simulink model "a7DOF"  (R2021a)
settings: Solver=VariableStepAuto  StartTime=0.0  StopTime=10.0  RelTol=1e-3
(part 1 of 2)
settings Model: Creator=RickyFang  LastModifiedBy=RickyFang

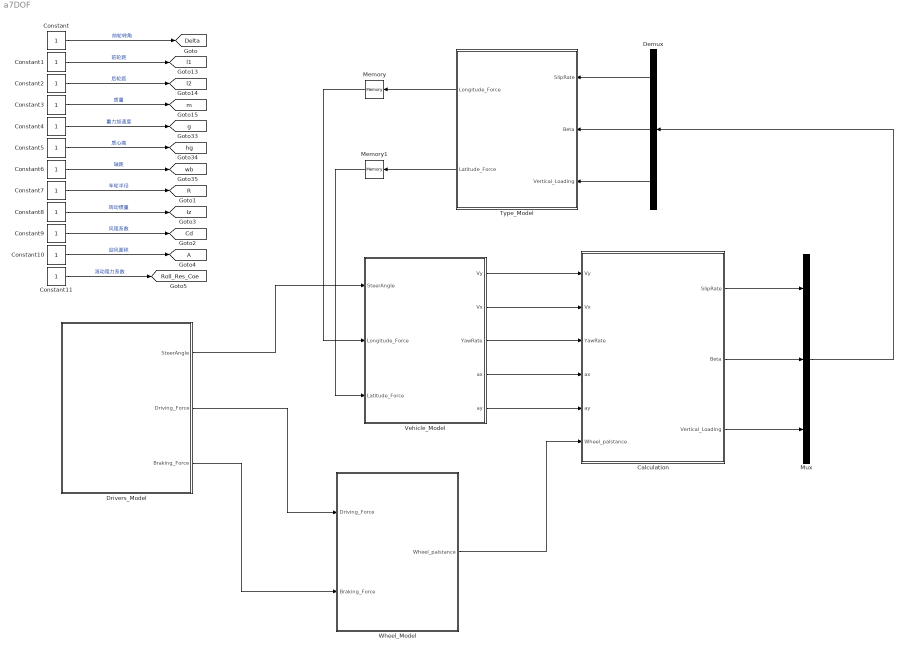
== system a7DOF ==
  Calculation : Subsystem
  Constant{,1..11} (12 alike) : Constant
  Demux : Demux  Outputs=3
  Drivers_Model : Subsystem
  Memory : Memory
  Memory1 : Memory
  Mux : Mux  Inputs=3
  Type_Model : Subsystem
  Vehicle_Model : Subsystem
  Wheel_Model : Subsystem
  tag scope: A=global, Cd=global, Delta=global, Iz=global, R=global, Roll_Res_Coe=global, g=global, hg=global, l1=global, l2=global, m=global, wb=global
  wires:
  Vehicle_Model/1(Vy) -> Calculation/1(Vy)
  Vehicle_Model/2(Vx) -> Calculation/2(Vx)
  Vehicle_Model/3(YawRate) -> Calculation/3(YawRate)
  Drivers_Model/1(SteerAngle) -> Vehicle_Model/1(SteerAngle)
  Drivers_Model/2(Driving_Force) -> Wheel_Model/1(Driving_Force)
  Drivers_Model/3(Braking_Force) -> Wheel_Model/2(Braking_Force)
  Calculation/2(Beta) -> Mux/2
  Calculation/1(SlipRate) -> Mux/1
  Demux/3 -> Type_Model/3(Vertical_Loading)
  Demux/2 -> Type_Model/2(Beta)
  Demux/1 -> Type_Model/1(SlipRate)
  Mux/1 -> Demux/1
  Calculation/3(Vertical_Loading) -> Mux/3
  Type_Model/2(Latitude_Force) -> Memory1/1
  Type_Model/1(Longitude_Force) -> Memory/1
  Memory/1 -> Vehicle_Model/2(Longitude_Force)
  Memory1/1 -> Vehicle_Model/3(Latitude_Force)
  Wheel_Model/1(Wheel_palstance) -> Calculation/6(Wheel_palstance)
  Vehicle_Model/4(ax) -> Calculation/4(ax)
  Vehicle_Model/5(ay) -> Calculation/5(ay)
  Constant/1 -> [Delta]  "前轮转角"
  Constant1/1 -> [l1]  "前轮距"
  Constant2/1 -> [l2]  "后轮距"
  Constant6/1 -> [wb]  "轴距"
  Constant5/1 -> [hg]  "质心高"
  Constant4/1 -> [g]  "重力加速度"
  Constant3/1 -> [m]  "质量"
  Constant7/1 -> [R]  "车轮半径"
  Constant8/1 -> [Iz]  "转动惯量"
  Constant9/1 -> [Cd]  "风阻系数"
  Constant10/1 -> [A]  "迎风面积"
  Constant11/1 -> [Roll_Res_Coe]  "滚动阻力系数"

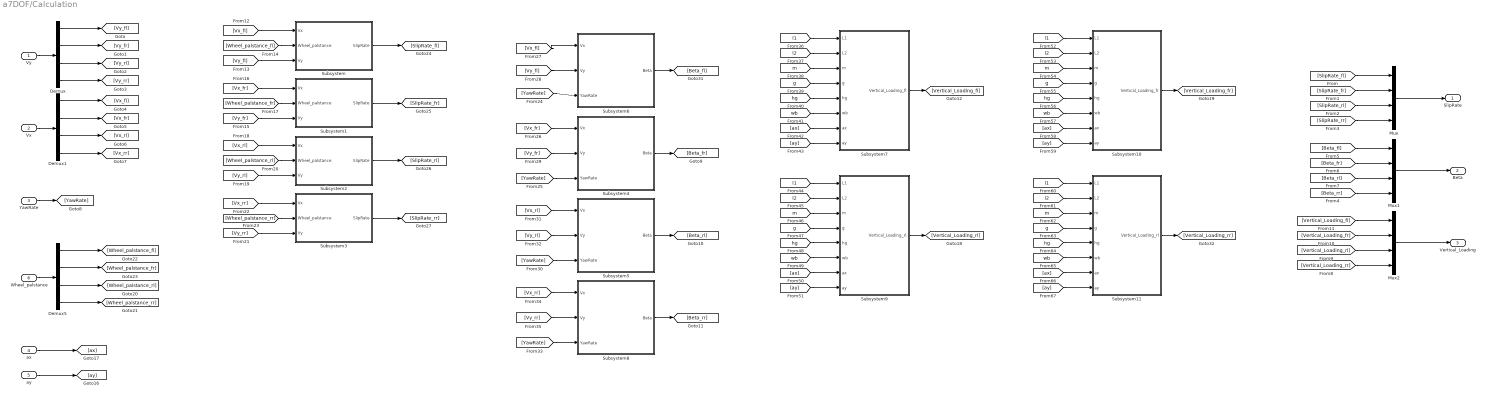
== system a7DOF/Calculation ==
  Vy : Inport
  Vx : Inport  Port=2
  YawRate : Inport  Port=3
  ax : Inport  Port=4
  ay : Inport  Port=5
  Wheel_palstance : Inport  Port=6
  Demux : Demux
  Demux1 : Demux
  Demux5 : Demux
  Mux : Mux
  Mux1 : Mux
  Mux2 : Mux
  Subsystem : Subsystem
  Subsystem1 : Subsystem
  Subsystem10 : Subsystem
  Subsystem11 : Subsystem
  Subsystem2 : Subsystem
  Subsystem3 : Subsystem
  Subsystem4 : Subsystem
  Subsystem5 : Subsystem
  Subsystem6 : Subsystem
  Subsystem7 : Subsystem
  Subsystem8 : Subsystem
  Subsystem9 : Subsystem
  SlipRate : Outport
  Beta : Outport  Port=2
  Vertical_Loading : Outport  Port=3
  wires:
  Vy/1 -> Demux/1
  Demux/1 -> [Vy_fl]
  Demux/2 -> [Vy_fr]
  Demux/3 -> [Vy_rl]
  Demux/4 -> [Vy_rr]
  Demux1/4 -> [Vx_rr]
  Demux1/3 -> [Vx_rl]
  Demux1/2 -> [Vx_fr]
  Demux1/1 -> [Vx_fl]
  Vx/1 -> Demux1/1
  YawRate/1 -> [YawRate]
  Demux5/4 -> [Wheel_palstance_rr]
  Demux5/3 -> [Wheel_palstance_rl]
  Demux5/2 -> [Wheel_palstance_fr]
  Demux5/1 -> [Wheel_palstance_fl]
  Wheel_palstance/1 -> Demux5/1
  Mux/1 -> SlipRate/1
  Mux1/1 -> Beta/1
  Mux2/1 -> Vertical_Loading/1
  [SlipRate_fl] -> Mux/1
  [SlipRate_fr] -> Mux/2
  [SlipRate_rl] -> Mux/3
  [SlipRate_rr] -> Mux/4
  [Beta_rr] -> Mux1/4
  [Beta_fl] -> Mux1/1
  [Beta_fr] -> Mux1/2
  [Beta_rl] -> Mux1/3
  [Vertical_Loading_rr] -> Mux2/4
  [Vertical_Loading_rl] -> Mux2/3
  [Vertical_Loading_fr] -> Mux2/2
  [Vertical_Loading_fl] -> Mux2/1
  [Vx_fl] -> Subsystem/1(Vx)
  [Vy_fl] -> Subsystem/3(Vy)
  [Wheel_palstance_fl] -> Subsystem/2(Wheel_palstance)
  [Vy_fr] -> Subsystem1/3(Vy)
  [Vx_fr] -> Subsystem1/1(Vx)
  [Wheel_palstance_fr] -> Subsystem1/2(Wheel_palstance)
  [Vx_rl] -> Subsystem2/1(Vx)
  [Vy_rl] -> Subsystem2/3(Vy)
  [Wheel_palstance_rl] -> Subsystem2/2(Wheel_palstance)
  [Vy_rr] -> Subsystem3/3(Vy)
  [Vx_rr] -> Subsystem3/1(Vx)
  [Wheel_palstance_rr] -> Subsystem3/2(Wheel_palstance)
  Subsystem/1(SlipRate) -> [SlipRate_fl]
  Subsystem1/1(SlipRate) -> [SlipRate_fr]
  Subsystem3/1(SlipRate) -> [SlipRate_rr]
  Subsystem2/1(SlipRate) -> [SlipRate_rl]
  [Vx_fl] -> Subsystem6/1(Vx)
  [Vy_fl] -> Subsystem6/2(Vy)
  Subsystem6/1(Beta) -> [Beta_fl]
  [l1] -> Subsystem7/1(L1)
  [l2] -> Subsystem7/2(L2)
  [m] -> Subsystem7/3(m)
  [g] -> Subsystem7/4(g)
  [hg] -> Subsystem7/5(hg)
  [wb] -> Subsystem7/6(wb)
  Subsystem7/1(Vertical_Loading_fl) -> [Vertical_Loading_fl]
  ay/1 -> [ay]
  ax/1 -> [ax]
  [ax] -> Subsystem7/7(ax)
  [ay] -> Subsystem7/8(ay)
  [ay] -> Subsystem9/8(ay)
  [ax] -> Subsystem9/7(ax)
  Subsystem9/1(Vertical_Loading_rl) -> [Vertical_Loading_rl]
  [wb] -> Subsystem9/6(wb)
  [hg] -> Subsystem9/5(hg)
  [g] -> Subsystem9/4(g)
  [m] -> Subsystem9/3(m)
  [l2] -> Subsystem9/2(L2)
  [l1] -> Subsystem9/1(L1)
  [l1] -> Subsystem10/1(L1)
  [l2] -> Subsystem10/2(L2)
  [m] -> Subsystem10/3(m)
  [g] -> Subsystem10/4(g)
  [hg] -> Subsystem10/5(hg)
  [wb] -> Subsystem10/6(wb)
  Subsystem10/1(Vertical_Loading_fr) -> [Vertical_Loading_fr]
  [ax] -> Subsystem10/7(ax)
  [ay] -> Subsystem10/8(ay)
  [ay] -> Subsystem11/8(ay)
  [ax] -> Subsystem11/7(ax)
  Subsystem11/1(Vertical_Loading_rl) -> [Vertical_Loading_rr]
  [wb] -> Subsystem11/6(wb)
  [hg] -> Subsystem11/5(hg)
  [g] -> Subsystem11/4(g)
  [m] -> Subsystem11/3(m)
  [l2] -> Subsystem11/2(L2)
  [l1] -> Subsystem11/1(L1)
  [YawRate] -> Subsystem6/3(YawRate)
  [YawRate] -> Subsystem4/3(YawRate)
  Subsystem4/1(Beta) -> [Beta_fr]
  [Vy_fr] -> Subsystem4/2(Vy)
  [Vx_fr] -> Subsystem4/1(Vx)
  [Vx_rl] -> Subsystem5/1(Vx)
  [Vy_rl] -> Subsystem5/2(Vy)
  Subsystem5/1(Beta) -> [Beta_rl]
  [YawRate] -> Subsystem5/3(YawRate)
  [YawRate] -> Subsystem8/3(YawRate)
  Subsystem8/1(Beta) -> [Beta_rr]
  [Vy_rr] -> Subsystem8/2(Vy)
  [Vx_rr] -> Subsystem8/1(Vx)

== system a7DOF/Drivers_Model ==
  SteerAngle : Outport
  Driving_Force : Outport  Port=2
  Braking_Force : Outport  Port=3
  wires:
  [Delta] -> SteerAngle/1

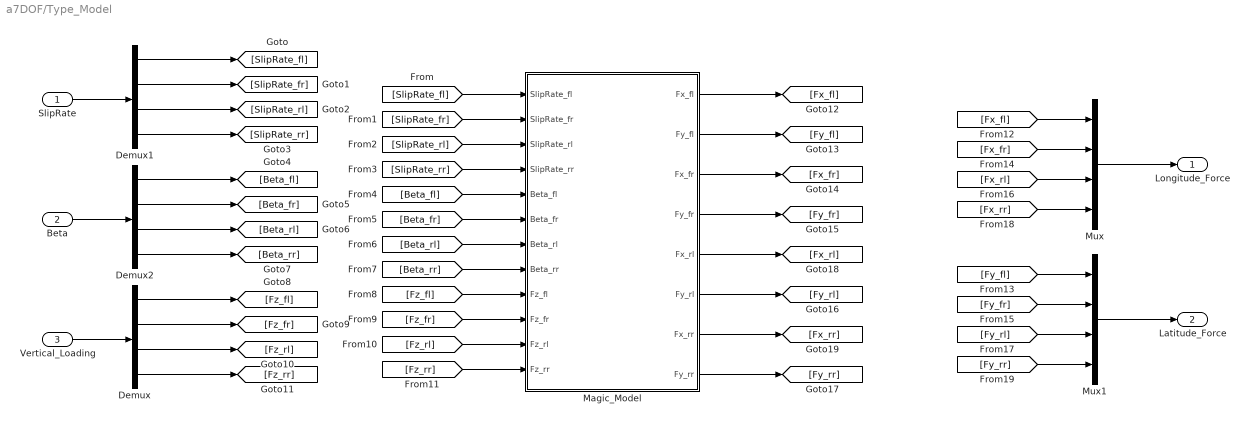
== system a7DOF/Type_Model ==
  SlipRate : Inport
  Beta : Inport  Port=2
  Vertical_Loading : Inport  Port=3
  Demux : Demux
  Demux1 : Demux
  Demux2 : Demux
  Magic_Model : Subsystem
  Mux : Mux
  Mux1 : Mux
  Longitude_Force : Outport
  Latitude_Force : Outport  Port=2
  wires:
  Vertical_Loading/1 -> Demux/1
  SlipRate/1 -> Demux1/1
  Beta/1 -> Demux2/1
  Demux1/1 -> [SlipRate_fl]
  Demux1/2 -> [SlipRate_fr]
  Demux1/3 -> [SlipRate_rl]
  Demux1/4 -> [SlipRate_rr]
  Demux2/4 -> [Beta_rr]
  Demux2/3 -> [Beta_rl]
  Demux2/2 -> [Beta_fr]
  Demux2/1 -> [Beta_fl]
  Demux/1 -> [Fz_fl]
  Demux/2 -> [Fz_fr]
  Demux/3 -> [Fz_rl]
  Demux/4 -> [Fz_rr]
  [SlipRate_fl] -> Magic_Model/1(SlipRate_fl)
  [SlipRate_fr] -> Magic_Model/2(SlipRate_fr)
  [SlipRate_rl] -> Magic_Model/3(SlipRate_rl)
  [SlipRate_rr] -> Magic_Model/4(SlipRate_rr)
  [Beta_fl] -> Magic_Model/5(Beta_fl)
  [Beta_fr] -> Magic_Model/6(Beta_fr)
  [Beta_rl] -> Magic_Model/7(Beta_rl)
  [Beta_rr] -> Magic_Model/8(Beta_rr)
  [Fz_fl] -> Magic_Model/9(Fz_fl)
  [Fz_fr] -> Magic_Model/10(Fz_fr)
  [Fz_rl] -> Magic_Model/11(Fz_rl)
  [Fz_rr] -> Magic_Model/12(Fz_rr)
  Magic_Model/1(Fx_fl) -> [Fx_fl]
  Magic_Model/2(Fy_fl) -> [Fy_fl]
  Magic_Model/3(Fx_fr) -> [Fx_fr]
  Magic_Model/4(Fy_fr) -> [Fy_fr]
  Magic_Model/6(Fy_rl) -> [Fy_rl]
  Magic_Model/8(Fy_rr) -> [Fy_rr]
  Magic_Model/5(Fx_rl) -> [Fx_rl]
  Magic_Model/7(Fx_rr) -> [Fx_rr]
  [Fx_fl] -> Mux/1
  [Fx_rr] -> Mux/4
  [Fx_fr] -> Mux/2
  [Fx_rl] -> Mux/3
  Mux/1 -> Longitude_Force/1
  [Fy_fl] -> Mux1/1
  [Fy_fr] -> Mux1/2
  [Fy_rr] -> Mux1/4
  [Fy_rl] -> Mux1/3
  Mux1/1 -> Latitude_Force/1

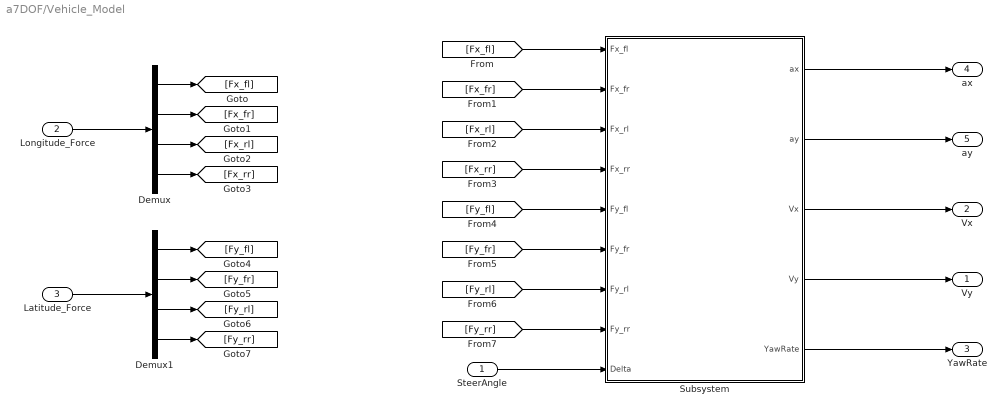
== system a7DOF/Vehicle_Model ==
  SteerAngle : Inport
  Longitude_Force : Inport  Port=2
  Latitude_Force : Inport  Port=3
  Demux : Demux
  Demux1 : Demux
  Subsystem : Subsystem
  Vy : Outport
  Vx : Outport  Port=2
  YawRate : Outport  Port=3
  ax : Outport  Port=4
  ay : Outport  Port=5
  wires:
  Longitude_Force/1 -> Demux/1
  Latitude_Force/1 -> Demux1/1
  Demux/1 -> [Fx_fl]
  Demux/2 -> [Fx_fr]
  Demux/3 -> [Fx_rl]
  Demux/4 -> [Fx_rr]
  Demux1/1 -> [Fy_fl]
  Demux1/2 -> [Fy_fr]
  Demux1/3 -> [Fy_rl]
  Demux1/4 -> [Fy_rr]
  [Fx_fl] -> Subsystem/1(Fx_fl)
  [Fx_fr] -> Subsystem/2(Fx_fr)
  [Fx_rl] -> Subsystem/3(Fx_rl)
  [Fx_rr] -> Subsystem/4(Fx_rr)
  [Fy_rr] -> Subsystem/8(Fy_rr)
  [Fy_rl] -> Subsystem/7(Fy_rl)
  [Fy_fr] -> Subsystem/6(Fy_fr)
  [Fy_fl] -> Subsystem/5(Fy_fl)
  SteerAngle/1 -> Subsystem/9(Delta)
  Subsystem/2(ay) -> ay/1
  Subsystem/4(Vy) -> Vy/1
  Subsystem/3(Vx) -> Vx/1
  Subsystem/1(ax) -> ax/1
  Subsystem/5(YawRate) -> YawRate/1

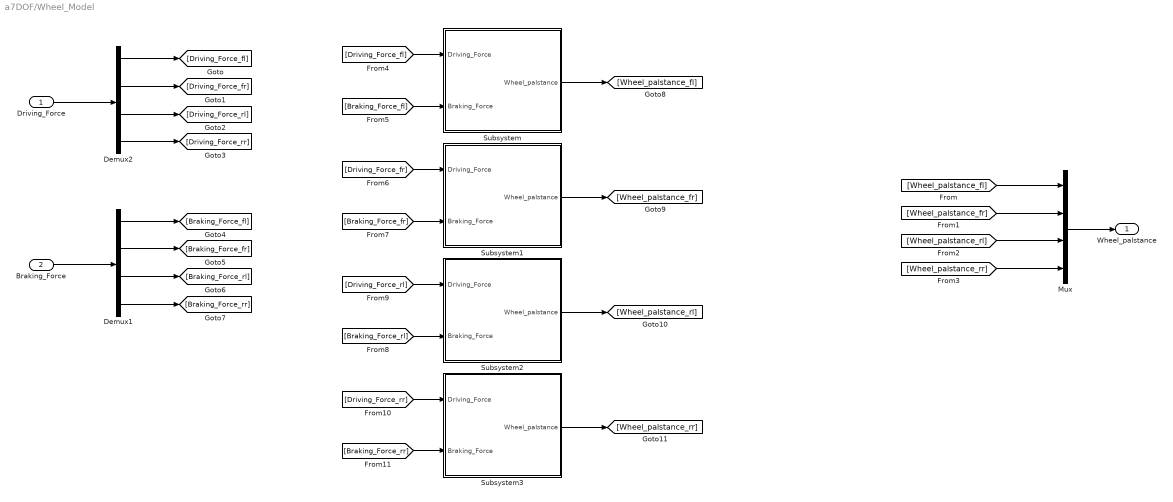
== system a7DOF/Wheel_Model ==
  Driving_Force : Inport
  Braking_Force : Inport  Port=2
  Demux1 : Demux
  Demux2 : Demux
  Mux : Mux
  Subsystem : Subsystem
  Subsystem1 : Subsystem
  Subsystem2 : Subsystem
  Subsystem3 : Subsystem
  Wheel_palstance : Outport
  wires:
  Driving_Force/1 -> Demux2/1
  Braking_Force/1 -> Demux1/1
  Demux2/1 -> [Driving_Force_fl]
  Demux2/2 -> [Driving_Force_fr]
  Demux2/3 -> [Driving_Force_rl]
  Demux2/4 -> [Driving_Force_rr]
  Demux1/1 -> [Braking_Force_fl]
  Demux1/2 -> [Braking_Force_fr]
  Demux1/3 -> [Braking_Force_rl]
  Demux1/4 -> [Braking_Force_rr]
  Mux/1 -> Wheel_palstance/1
  [Wheel_palstance_fr] -> Mux/2
  [Wheel_palstance_fl] -> Mux/1
  [Wheel_palstance_rl] -> Mux/3
  [Wheel_palstance_rr] -> Mux/4
  [Driving_Force_fl] -> Subsystem/1(Driving_Force)
  [Braking_Force_fl] -> Subsystem/2(Braking_Force)
  Subsystem/1(Wheel_palstance) -> [Wheel_palstance_fl]
  Subsystem1/1(Wheel_palstance) -> [Wheel_palstance_fr]
  [Driving_Force_fr] -> Subsystem1/1(Driving_Force)
  [Braking_Force_fr] -> Subsystem1/2(Braking_Force)
  [Driving_Force_rl] -> Subsystem2/1(Driving_Force)
  [Braking_Force_rl] -> Subsystem2/2(Braking_Force)
  Subsystem2/1(Wheel_palstance) -> [Wheel_palstance_rl]
  Subsystem3/1(Wheel_palstance) -> [Wheel_palstance_rr]
  [Braking_Force_rr] -> Subsystem3/2(Braking_Force)
  [Driving_Force_rr] -> Subsystem3/1(Driving_Force)

== system a7DOF/Calculation/Subsystem ==
  Vx : Inport
  Wheel_palstance : Inport  Port=2
  Vy : Inport  Port=3
  Abs : Abs
  Add : Sum
  Add1 : Sum  Inputs=+-
  Cos : Trigonometry  Operator=cos
  Cos1 : Trigonometry
  Divide : Product  Inputs=*/
  Max : MinMax  Function=max  Inputs=2
  Product : Product
  Product1 : Product
  Product2 : Product
  SlipRate : Outport
  wires:
  Wheel_palstance/1 -> Product/1
  [R] -> Product/2
  Divide/1 -> SlipRate/1
  [Delta] -> Cos/1
  Cos/1 -> Product1/1
  Vx/1 -> Product1/2
  Product1/1 -> Add/2
  Cos1/1 -> Product2/1
  [Delta] -> Cos1/1
  Vy/1 -> Product2/2
  Product2/1 -> Add/1
  Add/1 -> Max/1, Add1/1
  Product/1 -> Max/2, Add1/2
  Add1/1 -> Abs/1
  Abs/1 -> Divide/1
  Max/1 -> Divide/2

== system a7DOF/Calculation/Subsystem1 ==
  Vx : Inport
  Wheel_palstance : Inport  Port=2
  Vy : Inport  Port=3
  Abs : Abs
  Add : Sum
  Add1 : Sum  Inputs=+-
  Cos : Trigonometry  Operator=cos
  Cos1 : Trigonometry
  Divide : Product  Inputs=*/
  Max : MinMax  Function=max  Inputs=2
  Product : Product
  Product1 : Product
  Product2 : Product
  SlipRate : Outport
  wires:
  Max/1 -> Divide/2
  Abs/1 -> Divide/1
  Add1/1 -> Abs/1
  Product/1 -> Add1/2, Max/2
  Add/1 -> Add1/1, Max/1
  Product2/1 -> Add/1
  Vy/1 -> Product2/2
  [Delta] -> Cos1/1
  Cos1/1 -> Product2/1
  Product1/1 -> Add/2
  Vx/1 -> Product1/2
  Cos/1 -> Product1/1
  [Delta] -> Cos/1
  Divide/1 -> SlipRate/1
  [R] -> Product/2
  Wheel_palstance/1 -> Product/1

== system a7DOF/Calculation/Subsystem10 ==
  L1 : Inport
  L2 : Inport  Port=2
  m : Inport  Port=3
  g : Inport  Port=4
  hg : Inport  Port=5
  wb : Inport  Port=6
  ax : Inport  Port=7
  ay : Inport  Port=8
  Add : Sum  Inputs=+-+
  Subsystem : Subsystem
  Subsystem1 : Subsystem
  Subsystem2 : Subsystem
  Vertical_Loading_fr : Outport
  wires:
  m/1 -> Subsystem2/4(In4), Subsystem1/3(In3), Subsystem/3(In3)
  g/1 -> Subsystem/4(In4)
  hg/1 -> Subsystem2/5(In5), Subsystem1/4(In4)
  ax/1 -> Subsystem1/5(In5)
  L1/1 -> Subsystem2/1(In1), Subsystem1/1(In1), Subsystem/1(In1)
  L2/1 -> Subsystem2/2(In2), Subsystem2/3(In3), Subsystem1/2(In2), Subsystem/2(In2)
  wb/1 -> Subsystem2/6(In6)
  ay/1 -> Subsystem2/7(In7)
  Subsystem1/1(Out1) -> Add/2
  Subsystem/1(Out1) -> Add/1
  Subsystem2/1(Out1) -> Add/3
  Add/1 -> Vertical_Loading_fr/1

== system a7DOF/Calculation/Subsystem11 ==
  L1 : Inport
  L2 : Inport  Port=2
  m : Inport  Port=3
  g : Inport  Port=4
  hg : Inport  Port=5
  wb : Inport  Port=6
  ax : Inport  Port=7
  ay : Inport  Port=8
  Add : Sum  Inputs=+++
  Subsystem : Subsystem
  Subsystem1 : Subsystem
  Subsystem2 : Subsystem
  Vertical_Loading_rl : Outport
  wires:
  m/1 -> Subsystem2/4(In4), Subsystem1/3(In3), Subsystem/3(In3)
  g/1 -> Subsystem/4(In4)
  hg/1 -> Subsystem2/5(In5), Subsystem1/4(In4)
  ax/1 -> Subsystem1/5(In5)
  L1/1 -> Subsystem2/1(In1), Subsystem1/1(In1), Subsystem/1(In1)
  L2/1 -> Subsystem2/2(In2), Subsystem2/3(In3), Subsystem1/2(In2), Subsystem/2(In2)
  wb/1 -> Subsystem2/6(In6)
  ay/1 -> Subsystem2/7(In7)
  Subsystem1/1(Out1) -> Add/2
  Subsystem/1(Out1) -> Add/1
  Subsystem2/1(Out1) -> Add/3
  Add/1 -> Vertical_Loading_rl/1

== system a7DOF/Calculation/Subsystem2 ==
  Vx : Inport
  Wheel_palstance : Inport  Port=2
  Vy : Inport  Port=3
  Abs : Abs
  Add : Sum
  Add1 : Sum  Inputs=+-
  Cos : Trigonometry  Operator=cos
  Cos1 : Trigonometry
  Divide : Product  Inputs=*/
  Max : MinMax  Function=max  Inputs=2
  Product : Product
  Product1 : Product
  Product2 : Product
  SlipRate : Outport
  wires:
  Wheel_palstance/1 -> Product/1
  [R] -> Product/2
  Divide/1 -> SlipRate/1
  [Delta] -> Cos/1
  Cos/1 -> Product1/1
  Vx/1 -> Product1/2
  Product1/1 -> Add/2
  Cos1/1 -> Product2/1
  [Delta] -> Cos1/1
  Vy/1 -> Product2/2
  Product2/1 -> Add/1
  Add/1 -> Max/1, Add1/1
  Product/1 -> Max/2, Add1/2
  Add1/1 -> Abs/1
  Abs/1 -> Divide/1
  Max/1 -> Divide/2

== system a7DOF/Calculation/Subsystem3 ==
  Vx : Inport
  Wheel_palstance : Inport  Port=2
  Vy : Inport  Port=3
  Abs : Abs
  Add : Sum
  Add1 : Sum  Inputs=+-
  Cos : Trigonometry  Operator=cos
  Cos1 : Trigonometry
  Divide : Product  Inputs=*/
  Max : MinMax  Function=max  Inputs=2
  Product : Product
  Product1 : Product
  Product2 : Product
  SlipRate : Outport
  wires:
  Max/1 -> Divide/2
  Abs/1 -> Divide/1
  Add1/1 -> Abs/1
  Product/1 -> Add1/2, Max/2
  Add/1 -> Add1/1, Max/1
  Product2/1 -> Add/1
  Vy/1 -> Product2/2
  [Delta] -> Cos1/1
  Cos1/1 -> Product2/1
  Product1/1 -> Add/2
  Vx/1 -> Product1/2
  Cos/1 -> Product1/1
  [Delta] -> Cos/1
  Divide/1 -> SlipRate/1
  [R] -> Product/2
  Wheel_palstance/1 -> Product/1

== system a7DOF/Calculation/Subsystem4 ==
  Vx : Inport
  Vy : Inport  Port=2
  YawRate : Inport  Port=3
  Add : Sum
  Add1 : Sum
  Add2 : Sum  Inputs=+-
  Atan : Trigonometry  Operator=atan
  Divide : Product  Inputs=/*
  Gain : Gain  Gain=0.5
  Product : Product
  Product1 : Product
  YawRate1 : InportShadow  Port=3
  Beta : Outport
  wires:
  Add2/1 -> Beta/1
  Atan/1 -> Add2/2
  [Delta] -> Add2/1
  Divide/1 -> Atan/1
  Add/1 -> Divide/2
  Add1/1 -> Divide/1
  Product1/1 -> Add1/2
  Vx/1 -> Add1/1
  Gain/1 -> Product1/2
  [wb] -> Gain/1
  YawRate1/1 -> Product1/1
  Product/1 -> Add/2
  YawRate/1 -> Product/2
  [l1] -> Product/1
  Vy/1 -> Add/1

== system a7DOF/Calculation/Subsystem5 ==
  Vx : Inport
  Vy : Inport  Port=2
  YawRate : Inport  Port=3
  Add : Sum  Inputs=+-
  Add1 : Sum  Inputs=+-
  Atan : Trigonometry  Operator=atan
  Divide : Product  Inputs=/*
  Gain : Gain  Gain=0.5
  Gain1 : Gain  Gain=-1
  Product : Product
  Product1 : Product
  YawRate1 : InportShadow  Port=3
  Beta : Outport
  wires:
  Vy/1 -> Add/1
  [l2] -> Product/1
  YawRate/1 -> Product/2
  Product/1 -> Add/2
  YawRate1/1 -> Product1/1
  [wb] -> Gain/1
  Gain/1 -> Product1/2
  Vx/1 -> Add1/1
  Product1/1 -> Add1/2
  Add1/1 -> Divide/1
  Add/1 -> Divide/2
  Divide/1 -> Atan/1
  Gain1/1 -> Beta/1
  Atan/1 -> Gain1/1

== system a7DOF/Calculation/Subsystem6 ==
  Vx : Inport
  Vy : Inport  Port=2
  YawRate : Inport  Port=3
  Add : Sum
  Add1 : Sum  Inputs=+-
  Add2 : Sum  Inputs=+-
  Atan : Trigonometry  Operator=atan
  Divide : Product  Inputs=/*
  Gain : Gain  Gain=0.5
  Product : Product
  Product1 : Product
  YawRate1 : InportShadow  Port=3
  Beta : Outport
  wires:
  Vy/1 -> Add/1
  [l1] -> Product/1
  YawRate/1 -> Product/2
  Product/1 -> Add/2
  YawRate1/1 -> Product1/1
  [wb] -> Gain/1
  Gain/1 -> Product1/2
  Vx/1 -> Add1/1
  Product1/1 -> Add1/2
  Add1/1 -> Divide/1
  Add/1 -> Divide/2
  Divide/1 -> Atan/1
  [Delta] -> Add2/1
  Atan/1 -> Add2/2
  Add2/1 -> Beta/1

== system a7DOF/Calculation/Subsystem7 ==
  L1 : Inport
  L2 : Inport  Port=2
  m : Inport  Port=3
  g : Inport  Port=4
  hg : Inport  Port=5
  wb : Inport  Port=6
  ax : Inport  Port=7
  ay : Inport  Port=8
  Add : Sum  Inputs=+--
  Subsystem : Subsystem
  Subsystem1 : Subsystem
  Subsystem2 : Subsystem
  Vertical_Loading_fl : Outport
  wires:
  m/1 -> Subsystem2/4(In4), Subsystem1/3(In3), Subsystem/3(In3)
  g/1 -> Subsystem/4(In4)
  hg/1 -> Subsystem2/5(In5), Subsystem1/4(In4)
  ax/1 -> Subsystem1/5(In5)
  L1/1 -> Subsystem2/1(In1), Subsystem1/1(In1), Subsystem/1(In1)
  L2/1 -> Subsystem2/2(In2), Subsystem2/3(In3), Subsystem1/2(In2), Subsystem/2(In2)
  wb/1 -> Subsystem2/6(In6)
  ay/1 -> Subsystem2/7(In7)
  Subsystem1/1(Out1) -> Add/2
  Subsystem/1(Out1) -> Add/1
  Subsystem2/1(Out1) -> Add/3
  Add/1 -> Vertical_Loading_fl/1

== system a7DOF/Calculation/Subsystem8 ==
  Vx : Inport
  Vy : Inport  Port=2
  YawRate : Inport  Port=3
  Add : Sum  Inputs=+-
  Add1 : Sum
  Atan : Trigonometry  Operator=atan
  Divide : Product  Inputs=/*
  Gain : Gain  Gain=0.5
  Gain1 : Gain  Gain=-1
  Product : Product
  Product1 : Product
  YawRate1 : InportShadow  Port=3
  Beta : Outport
  wires:
  Atan/1 -> Gain1/1
  Gain1/1 -> Beta/1
  Divide/1 -> Atan/1
  Add/1 -> Divide/2
  Add1/1 -> Divide/1
  Product1/1 -> Add1/2
  Vx/1 -> Add1/1
  Gain/1 -> Product1/2
  [wb] -> Gain/1
  YawRate1/1 -> Product1/1
  Product/1 -> Add/2
  YawRate/1 -> Product/2
  [l2] -> Product/1
  Vy/1 -> Add/1

== system a7DOF/Calculation/Subsystem9 ==
  L1 : Inport
  L2 : Inport  Port=2
  m : Inport  Port=3
  g : Inport  Port=4
  hg : Inport  Port=5
  wb : Inport  Port=6
  ax : Inport  Port=7
  ay : Inport  Port=8
  Add : Sum  Inputs=++-
  Subsystem : Subsystem
  Subsystem1 : Subsystem
  Subsystem2 : Subsystem
  Vertical_Loading_rl : Outport
  wires:
  Add/1 -> Vertical_Loading_rl/1
  Subsystem2/1(Out1) -> Add/3
  Subsystem/1(Out1) -> Add/1
  Subsystem1/1(Out1) -> Add/2
  ay/1 -> Subsystem2/7(In7)
  wb/1 -> Subsystem2/6(In6)
  L2/1 -> Subsystem/2(In2), Subsystem1/2(In2), Subsystem2/3(In3), Subsystem2/2(In2)
  L1/1 -> Subsystem/1(In1), Subsystem1/1(In1), Subsystem2/1(In1)
  ax/1 -> Subsystem1/5(In5)
  hg/1 -> Subsystem1/4(In4), Subsystem2/5(In5)
  g/1 -> Subsystem/4(In4)
  m/1 -> Subsystem/3(In3), Subsystem1/3(In3), Subsystem2/4(In4)

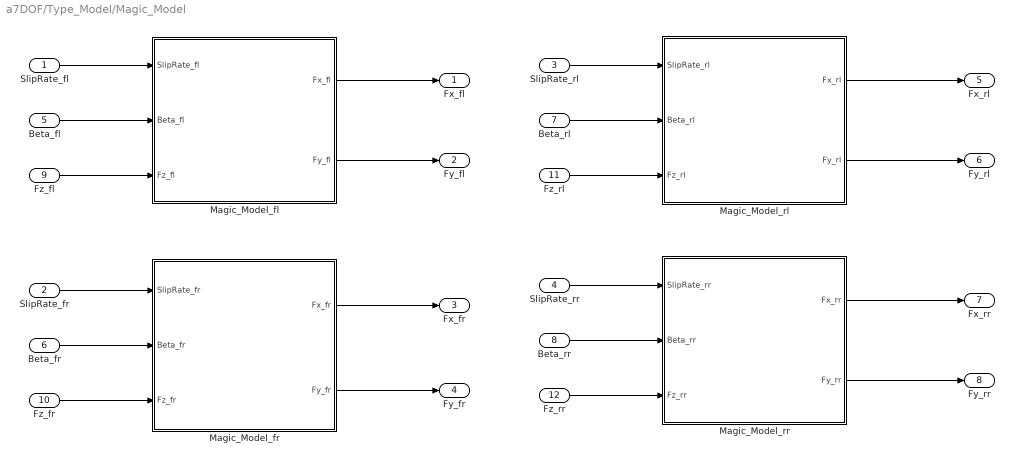
== system a7DOF/Type_Model/Magic_Model ==
  SlipRate_fl : Inport
  SlipRate_fr : Inport  Port=2
  SlipRate_rl : Inport  Port=3
  SlipRate_rr : Inport  Port=4
  Beta_fl : Inport  Port=5
  Beta_fr : Inport  Port=6
  Beta_rl : Inport  Port=7
  Beta_rr : Inport  Port=8
  Fz_fl : Inport  Port=9
  Fz_fr : Inport  Port=10
  Fz_rl : Inport  Port=11
  Fz_rr : Inport  Port=12
  Magic_Model_fl : Subsystem
  Magic_Model_fr : Subsystem
  Magic_Model_rl : Subsystem
  Magic_Model_rr : Subsystem
  Fx_fl : Outport
  Fy_fl : Outport  Port=2
  Fx_fr : Outport  Port=3
  Fy_fr : Outport  Port=4
  Fx_rl : Outport  Port=5
  Fy_rl : Outport  Port=6
  Fx_rr : Outport  Port=7
  Fy_rr : Outport  Port=8
  wires:
  SlipRate_fl/1 -> Magic_Model_fl/1(SlipRate_fl)
  Beta_fl/1 -> Magic_Model_fl/2(Beta_fl)
  Fz_fl/1 -> Magic_Model_fl/3(Fz_fl)
  Magic_Model_fl/1(Fx_fl) -> Fx_fl/1
  Magic_Model_fl/2(Fy_fl) -> Fy_fl/1
  SlipRate_fr/1 -> Magic_Model_fr/1(SlipRate_fr)
  Beta_fr/1 -> Magic_Model_fr/2(Beta_fr)
  Fz_fr/1 -> Magic_Model_fr/3(Fz_fr)
  Magic_Model_fr/1(Fx_fr) -> Fx_fr/1
  Magic_Model_fr/2(Fy_fr) -> Fy_fr/1
  SlipRate_rl/1 -> Magic_Model_rl/1(SlipRate_rl)
  Beta_rl/1 -> Magic_Model_rl/2(Beta_rl)
  Fz_rl/1 -> Magic_Model_rl/3(Fz_rl)
  Magic_Model_rl/1(Fx_rl) -> Fx_rl/1
  Magic_Model_rl/2(Fy_rl) -> Fy_rl/1
  SlipRate_rr/1 -> Magic_Model_rr/1(SlipRate_rr)
  Beta_rr/1 -> Magic_Model_rr/2(Beta_rr)
  Fz_rr/1 -> Magic_Model_rr/3(Fz_rr)
  Magic_Model_rr/1(Fx_rr) -> Fx_rr/1
  Magic_Model_rr/2(Fy_rr) -> Fy_rr/1

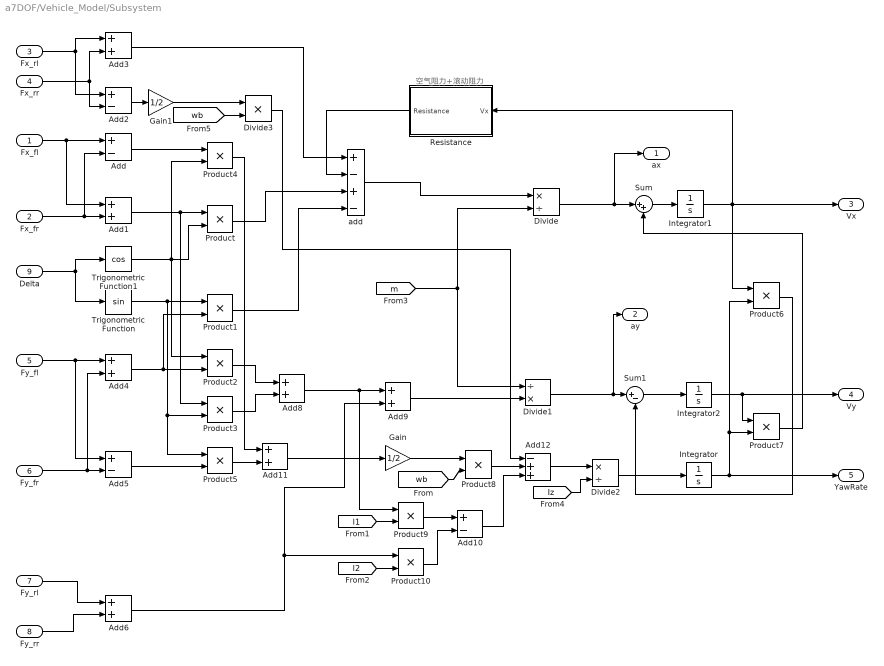
== system a7DOF/Vehicle_Model/Subsystem ==
  note: 空气阻力+滚动阻力
  Fx_fl : Inport
  Fx_fr : Inport  Port=2
  Fx_rl : Inport  Port=3
  Fx_rr : Inport  Port=4
  Fy_fl : Inport  Port=5
  Fy_fr : Inport  Port=6
  Fy_rl : Inport  Port=7
  Fy_rr : Inport  Port=8
  Delta : Inport  Port=9
  Add{,2,5,10} (4 alike) : Sum  Inputs=+-
  Add{1,3..4,6,8..9,11} (7 alike) : Sum
  Add12 : Sum  Inputs=-++
  Divide : Product  Inputs=*/
  Divide1 : Product  Inputs=/*
  Divide2 : Product  Inputs=*/
  Divide3 : Product  Inputs=**
  Gain : Gain  Gain=1/2
  Gain1 : Gain  Gain=1/2
  Integrator : Integrator
  Integrator1 : Integrator  InitialCondition=eps  UpperSaturationLimit=35  LowerSaturationLimit=0
  Integrator2 : Integrator
  Product{,1..7} (8 alike) : Product  RndMeth=Zero
  Product10 : Product
  Product8 : Product
  Product9 : Product
  Resistance : Subsystem
  Sum : Sum  Inputs=|++
  Sum1 : Sum  Inputs=|+-
  Trigonometric Function : Trigonometry
  Trigonometric Function1 : Trigonometry  Operator=cos
  add : Sum  Inputs=+-+-
  ax : Outport
  ay : Outport  Port=2
  Vx : Outport  Port=3
  Vy : Outport  Port=4
  YawRate : Outport  Port=5
  wires:
  Sum1/1 -> Integrator2/1
  Add9/1 -> Divide1/2
  Fx_fr/1 -> Add/2, Add1/2
  Sum/1 -> Integrator1/1
  Resistance/1(Resistance) -> add/2
  add/1 -> Divide/1
  Product2/1 -> Add8/1
  Add2/1 -> Gain1/1
  Product8/1 -> Add12/2
  Add8/1 -> Product9/1, Add9/1
  Add/1 -> Product4/1
  Integrator2/1 -> Product7/1, Vy/1
  Product3/1 -> Add8/2
  Product5/1 -> Add11/2
  Add6/1 -> Product10/1, Add9/2
  [m] -> Divide1/1, Divide/2
  Fx_rr/1 -> Add3/2, Add2/2
  Add4/1 -> Product1/2, Product2/2
  Product9/1 -> Add10/1
  Fy_fl/1 -> Add4/1, Add5/1
  Trigonometric Function/1 -> Product1/1, Product3/2, Product5/1
  Divide/1 -> Sum/1, ax/1
  Add3/1 -> add/1
  Fx_fl/1 -> Add/1, Add1/1
  Divide2/1 -> Integrator/1
  Add1/1 -> Product/1, Product3/1
  Integrator1/1 -> Product6/1, Vx/1, Resistance/1("Vx ")
  Delta/1 -> Trigonometric Function/1, Trigonometric Function1/1
  Fx_rl/1 -> Add2/1, Add3/1
  Fy_rl/1 -> Add6/1
  Trigonometric Function1/1 -> Product/2, Product2/1, Product4/2
  Product1/1 -> add/4
  Product10/1 -> Add10/2
  Product/1 -> add/3
  Add10/1 -> Add12/3
  Fy_rr/1 -> Add6/2
  Product4/1 -> Add11/1
  Product6/1 -> Sum1/2
  Divide1/1 -> Sum1/1, ay/1
  Product7/1 -> Sum/2
  Add12/1 -> Divide2/1
  Fy_fr/1 -> Add5/2, Add4/2
  Integrator/1 -> Product6/2, Product7/2, YawRate/1
  Add5/1 -> Product5/2
  [wb] -> Product8/2
  Add11/1 -> Gain/1
  Gain/1 -> Product8/1
  [l1] -> Product9/2
  [l2] -> Product10/2
  [Iz] -> Divide2/2
  Divide3/1 -> Add12/1
  Gain1/1 -> Divide3/1
  [wb] -> Divide3/2

== system a7DOF/Wheel_Model/Subsystem ==
  Driving_Force : Inport
  Braking_Force : Inport  Port=2
  Add : Sum  Inputs=+-
  Divide : Product  Inputs=*//
  Integrator : Integrator
  Wheel_palstance : Outport
  wires:
  Divide/1 -> Integrator/1
  Braking_Force/1 -> Add/2
  Add/1 -> Divide/1
  [m] -> Divide/3
  [R] -> Divide/2
  Driving_Force/1 -> Add/1
  Integrator/1 -> Wheel_palstance/1

== system a7DOF/Wheel_Model/Subsystem1 ==
  Driving_Force : Inport
  Braking_Force : Inport  Port=2
  Add : Sum  Inputs=+-
  Divide : Product  Inputs=*//
  Integrator : Integrator
  Wheel_palstance : Outport
  wires:
  Integrator/1 -> Wheel_palstance/1
  Driving_Force/1 -> Add/1
  [R] -> Divide/2
  [m] -> Divide/3
  Add/1 -> Divide/1
  Braking_Force/1 -> Add/2
  Divide/1 -> Integrator/1

== system a7DOF/Wheel_Model/Subsystem2 ==
  Driving_Force : Inport
  Braking_Force : Inport  Port=2
  Add : Sum  Inputs=+-
  Divide : Product  Inputs=*//
  Integrator : Integrator
  Wheel_palstance : Outport
  wires:
  Divide/1 -> Integrator/1
  Braking_Force/1 -> Add/2
  Add/1 -> Divide/1
  [m] -> Divide/3
  [R] -> Divide/2
  Driving_Force/1 -> Add/1
  Integrator/1 -> Wheel_palstance/1

== system a7DOF/Wheel_Model/Subsystem3 ==
  Driving_Force : Inport
  Braking_Force : Inport  Port=2
  Add : Sum  Inputs=+-
  Divide : Product  Inputs=*//
  Integrator : Integrator
  Wheel_palstance : Outport
  wires:
  Integrator/1 -> Wheel_palstance/1
  Driving_Force/1 -> Add/1
  [R] -> Divide/2
  [m] -> Divide/3
  Add/1 -> Divide/1
  Braking_Force/1 -> Add/2
  Divide/1 -> Integrator/1

== system a7DOF/Calculation/Subsystem10/Subsystem ==
  In1 : Inport
  In2 : Inport  Port=2
  In3 : Inport  Port=3
  In4 : Inport  Port=4
  Add : Sum
  Divide : Product  Inputs=***/
  Gain : Gain  Gain=2
  Out1 : Outport
  wires:
  In1/1 -> Add/1
  Add/1 -> Gain/1
  In2/1 -> Divide/1, Add/2
  Gain/1 -> Divide/4
  In3/1 -> Divide/2
  Divide/1 -> Out1/1
  In4/1 -> Divide/3

== system a7DOF/Calculation/Subsystem10/Subsystem1 ==
  In1 : Inport
  In2 : Inport  Port=2
  In3 : Inport  Port=3
  In4 : Inport  Port=4
  In5 : Inport  Port=5
  Add : Sum
  Divide : Product  Inputs=***/
  Gain : Gain  Gain=2
  Out1 : Outport
  wires:
  Divide/1 -> Out1/1
  In4/1 -> Divide/3
  Gain/1 -> Divide/4
  In3/1 -> Divide/1
  In1/1 -> Add/1
  Add/1 -> Gain/1
  In5/1 -> Divide/2
  In2/1 -> Add/2

== system a7DOF/Calculation/Subsystem10/Subsystem2 ==
  In1 : Inport
  In2 : Inport  Port=2
  In3 : Inport  Port=3
  In4 : Inport  Port=4
  In5 : Inport  Port=5
  In6 : Inport  Port=6
  In7 : Inport  Port=7
  Add : Sum
  Divide : Product  Inputs=****//
  Gain : Gain  Gain=2
  Out1 : Outport
  wires:
  In6/1 -> Divide/5
  In3/1 -> Divide/4
  Add/1 -> Gain/1
  Divide/1 -> Out1/1
  In2/1 -> Add/2
  In1/1 -> Add/1
  Gain/1 -> Divide/6
  In4/1 -> Divide/1
  In7/1 -> Divide/2
  In5/1 -> Divide/3

== system a7DOF/Calculation/Subsystem11/Subsystem ==
  In1 : Inport
  In2 : Inport  Port=2
  In3 : Inport  Port=3
  In4 : Inport  Port=4
  Add : Sum
  Divide : Product  Inputs=***/
  Gain : Gain  Gain=2
  Out1 : Outport
  wires:
  In2/1 -> Add/1
  Add/1 -> Gain/1
  In1/1 -> Divide/1, Add/2
  Gain/1 -> Divide/4
  In3/1 -> Divide/2
  Divide/1 -> Out1/1
  In4/1 -> Divide/3

== system a7DOF/Calculation/Subsystem11/Subsystem1 ==
  In1 : Inport
  In2 : Inport  Port=2
  In3 : Inport  Port=3
  In4 : Inport  Port=4
  In5 : Inport  Port=5
  Add : Sum
  Divide : Product  Inputs=***/
  Gain : Gain  Gain=2
  Out1 : Outport
  wires:
  Divide/1 -> Out1/1
  In4/1 -> Divide/3
  Gain/1 -> Divide/4
  In3/1 -> Divide/1
  In1/1 -> Add/1
  Add/1 -> Gain/1
  In5/1 -> Divide/2
  In2/1 -> Add/2

== system a7DOF/Calculation/Subsystem11/Subsystem2 ==
  In1 : Inport
  In2 : Inport  Port=2
  In3 : Inport  Port=3
  In4 : Inport  Port=4
  In5 : Inport  Port=5
  In6 : Inport  Port=6
  In7 : Inport  Port=7
  Add : Sum
  Divide : Product  Inputs=****//
  Gain : Gain  Gain=2
  Out1 : Outport
  wires:
  In6/1 -> Divide/5
  In3/1 -> Divide/4
  Add/1 -> Gain/1
  Divide/1 -> Out1/1
  In1/1 -> Add/2
  In2/1 -> Add/1
  Gain/1 -> Divide/6
  In4/1 -> Divide/1
  In7/1 -> Divide/2
  In5/1 -> Divide/3

== system a7DOF/Calculation/Subsystem7/Subsystem ==
  In1 : Inport
  In2 : Inport  Port=2
  In3 : Inport  Port=3
  In4 : Inport  Port=4
  Add : Sum
  Divide : Product  Inputs=***/
  Gain : Gain  Gain=2
  Out1 : Outport
  wires:
  In1/1 -> Add/1
  Add/1 -> Gain/1
  In2/1 -> Divide/1, Add/2
  Gain/1 -> Divide/4
  In3/1 -> Divide/2
  Divide/1 -> Out1/1
  In4/1 -> Divide/3

== system a7DOF/Calculation/Subsystem7/Subsystem1 ==
  In1 : Inport
  In2 : Inport  Port=2
  In3 : Inport  Port=3
  In4 : Inport  Port=4
  In5 : Inport  Port=5
  Add : Sum
  Divide : Product  Inputs=***/
  Gain : Gain  Gain=2
  Out1 : Outport
  wires:
  Divide/1 -> Out1/1
  In4/1 -> Divide/3
  Gain/1 -> Divide/4
  In3/1 -> Divide/1
  In1/1 -> Add/1
  Add/1 -> Gain/1
  In5/1 -> Divide/2
  In2/1 -> Add/2

== system a7DOF/Calculation/Subsystem7/Subsystem2 ==
  In1 : Inport
  In2 : Inport  Port=2
  In3 : Inport  Port=3
  In4 : Inport  Port=4
  In5 : Inport  Port=5
  In6 : Inport  Port=6
  In7 : Inport  Port=7
  Add : Sum
  Divide : Product  Inputs=****//
  Gain : Gain  Gain=2
  Out1 : Outport
  wires:
  In6/1 -> Divide/5
  In3/1 -> Divide/4
  Add/1 -> Gain/1
  Divide/1 -> Out1/1
  In2/1 -> Add/2
  In1/1 -> Add/1
  Gain/1 -> Divide/6
  In4/1 -> Divide/1
  In7/1 -> Divide/2
  In5/1 -> Divide/3

== system a7DOF/Calculation/Subsystem9/Subsystem ==
  In1 : Inport
  In2 : Inport  Port=2
  In3 : Inport  Port=3
  In4 : Inport  Port=4
  Add : Sum
  Divide : Product  Inputs=***/
  Gain : Gain  Gain=2
  Out1 : Outport
  wires:
  In4/1 -> Divide/3
  Divide/1 -> Out1/1
  In3/1 -> Divide/2
  Gain/1 -> Divide/4
  In1/1 -> Add/2, Divide/1
  Add/1 -> Gain/1
  In2/1 -> Add/1

== system a7DOF/Calculation/Subsystem9/Subsystem1 ==
  In1 : Inport
  In2 : Inport  Port=2
  In3 : Inport  Port=3
  In4 : Inport  Port=4
  In5 : Inport  Port=5
  Add : Sum
  Divide : Product  Inputs=***/
  Gain : Gain  Gain=2
  Out1 : Outport
  wires:
  In2/1 -> Add/2
  In5/1 -> Divide/2
  Add/1 -> Gain/1
  In1/1 -> Add/1
  In3/1 -> Divide/1
  Gain/1 -> Divide/4
  In4/1 -> Divide/3
  Divide/1 -> Out1/1

== system a7DOF/Calculation/Subsystem9/Subsystem2 ==
  In1 : Inport
  In2 : Inport  Port=2
  In3 : Inport  Port=3
  In4 : Inport  Port=4
  In5 : Inport  Port=5
  In6 : Inport  Port=6
  In7 : Inport  Port=7
  Add : Sum
  Divide : Product  Inputs=****//
  Gain : Gain  Gain=2
  Out1 : Outport
  wires:
  In5/1 -> Divide/3
  In7/1 -> Divide/2
  In4/1 -> Divide/1
  Gain/1 -> Divide/6
  In2/1 -> Add/1
  In1/1 -> Add/2
  Divide/1 -> Out1/1
  Add/1 -> Gain/1
  In3/1 -> Divide/4
  In6/1 -> Divide/5

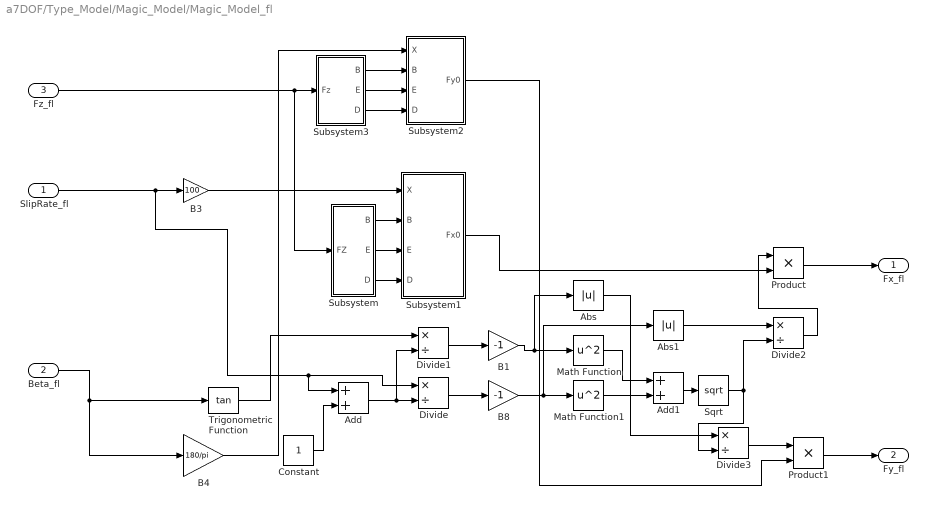
== system a7DOF/Type_Model/Magic_Model/Magic_Model_fl ==
  SlipRate_fl : Inport
  Beta_fl : Inport  Port=2
  Fz_fl : Inport  Port=3
  Abs : Abs
  Abs1 : Abs
  Add : Sum
  Add1 : Sum
  B1 : Gain  Gain=-1
  B3 : Gain  Gain=100
  B4 : Gain  Gain=180/pi
  B8 : Gain  Gain=-1
  Constant : Constant
  Divide{,1..3} (4 alike) : Product  Inputs=*/
  Math Function : Math  Operator=square  SignedPower=on  SaturateOnIntegerOverflow=on
  Math Function1 : Math  Operator=square  SignedPower=on  SaturateOnIntegerOverflow=on
  Product : Product  RndMeth=Zero
  Product1 : Product  RndMeth=Zero
  Sqrt : Sqrt  SaturateOnIntegerOverflow=on
  Subsystem : Subsystem
  Subsystem1 : Subsystem
  Subsystem2 : Subsystem
  Subsystem3 : Subsystem
  Trigonometric Function : Trigonometry  Operator=tan
  Fx_fl : Outport
  Fy_fl : Outport  Port=2
  wires:
  SlipRate_fl/1 -> Divide/1, Add/1, B3/1
  B4/1 -> Subsystem2/1("X ")
  Beta_fl/1 -> B4/1, Trigonometric Function/1
  Abs1/1 -> Divide2/1
  Math Function1/1 -> Add1/2
  Subsystem/3("D ") -> Subsystem1/4(D)
  Subsystem3/2("E ") -> Subsystem2/3(E)
  Fz_fl/1 -> Subsystem/1(FZ), Subsystem3/1("Fz ")
  Subsystem3/1("B ") -> Subsystem2/2(B)
  B8/1 -> Abs1/1, Math Function1/1
  Divide1/1 -> B1/1
  Subsystem3/3("D ") -> Subsystem2/4(D)
  Subsystem/1("B ") -> Subsystem1/2(B)
  Product1/1 -> Fy_fl/1
  Subsystem2/1(Fy0) -> Product1/2
  Divide3/1 -> Product1/1
  B1/1 -> Abs/1, Math Function/1
  Divide/1 -> B8/1
  Subsystem1/1(Fx0) -> Product/2
  Subsystem/2(E) -> Subsystem1/3(E)
  Math Function/1 -> Add1/1
  Add/1 -> Divide1/2, Divide/2
  Add1/1 -> Sqrt/1
  Trigonometric Function/1 -> Divide1/1
  Sqrt/1 -> Divide3/2, Divide2/2
  Abs/1 -> Divide3/1
  B3/1 -> Subsystem1/1(X)
  Divide2/1 -> Product/1
  Product/1 -> Fx_fl/1
  Constant/1 -> Add/2

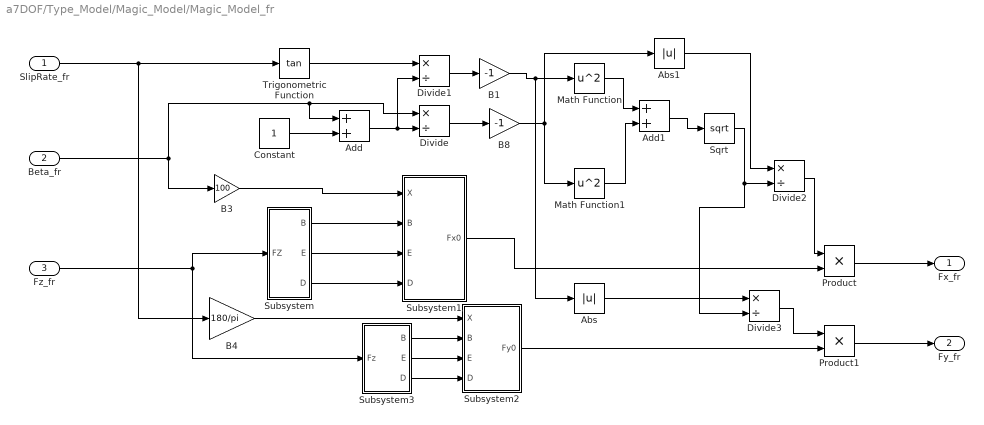
== system a7DOF/Type_Model/Magic_Model/Magic_Model_fr ==
  SlipRate_fr : Inport
  Beta_fr : Inport  Port=2
  Fz_fr : Inport  Port=3
  Abs : Abs
  Abs1 : Abs
  Add : Sum
  Add1 : Sum
  B1 : Gain  Gain=-1
  B3 : Gain  Gain=100
  B4 : Gain  Gain=180/pi
  B8 : Gain  Gain=-1
  Constant : Constant
  Divide{,1..3} (4 alike) : Product  Inputs=*/
  Math Function : Math  Operator=square  SignedPower=on  SaturateOnIntegerOverflow=on
  Math Function1 : Math  Operator=square  SignedPower=on  SaturateOnIntegerOverflow=on
  Product : Product  RndMeth=Zero
  Product1 : Product  RndMeth=Zero
  Sqrt : Sqrt  SaturateOnIntegerOverflow=on
  Subsystem : Subsystem
  Subsystem1 : Subsystem
  Subsystem2 : Subsystem
  Subsystem3 : Subsystem
  Trigonometric Function : Trigonometry  Operator=tan
  Fx_fr : Outport
  Fy_fr : Outport  Port=2
  wires:
  B3/1 -> Subsystem1/1(X)
  Add/1 -> Divide1/2, Divide/2
  Subsystem1/1(Fx0) -> Product/2
  SlipRate_fr/1 -> B4/1, Trigonometric Function/1
  Subsystem3/3("D ") -> Subsystem2/4(D)
  Abs/1 -> Divide3/1
  Subsystem/2(E) -> Subsystem1/3(E)
  Subsystem3/2("E ") -> Subsystem2/3(E)
  Divide3/1 -> Product1/1
  Subsystem/1("B ") -> Subsystem1/2(B)
  Abs1/1 -> Divide2/1
  Trigonometric Function/1 -> Divide1/1
  Product/1 -> Fx_fr/1
  Subsystem/3("D ") -> Subsystem1/4(D)
  Subsystem3/1("B ") -> Subsystem2/2(B)
  Beta_fr/1 -> B3/1, Add/1, Divide/1
  B8/1 -> Abs1/1, Math Function1/1
  Divide1/1 -> B1/1
  Divide2/1 -> Product/1
  Subsystem2/1(Fy0) -> Product1/2
  Fz_fr/1 -> Subsystem/1(FZ), Subsystem3/1("Fz ")
  Constant/1 -> Add/2
  B1/1 -> Abs/1, Math Function/1
  Sqrt/1 -> Divide3/2, Divide2/2
  Add1/1 -> Sqrt/1
  Math Function1/1 -> Add1/2
  Product1/1 -> Fy_fr/1
  B4/1 -> Subsystem2/1("X ")
  Math Function/1 -> Add1/1
  Divide/1 -> B8/1

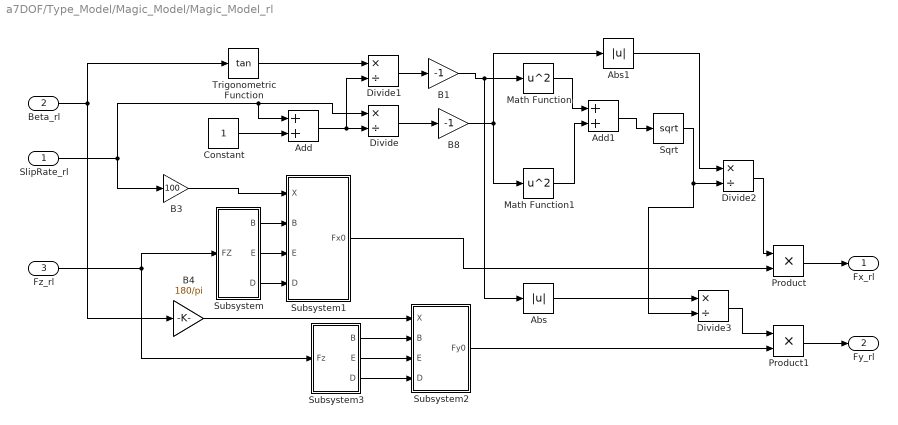
== system a7DOF/Type_Model/Magic_Model/Magic_Model_rl ==
  SlipRate_rl : Inport
  Beta_rl : Inport  Port=2
  Fz_rl : Inport  Port=3
  Abs : Abs
  Abs1 : Abs
  Add : Sum
  Add1 : Sum
  B1 : Gain  Gain=-1
  B3 : Gain  Gain=100
  B4 : Gain  Gain=180/pi
  B8 : Gain  Gain=-1
  Constant : Constant
  Divide{,1..3} (4 alike) : Product  Inputs=*/
  Math Function : Math  Operator=square  SignedPower=on  SaturateOnIntegerOverflow=on
  Math Function1 : Math  Operator=square  SignedPower=on  SaturateOnIntegerOverflow=on
  Product : Product  RndMeth=Zero
  Product1 : Product  RndMeth=Zero
  Sqrt : Sqrt  SaturateOnIntegerOverflow=on
  Subsystem : Subsystem
  Subsystem1 : Subsystem
  Subsystem2 : Subsystem
  Subsystem3 : Subsystem
  Trigonometric Function : Trigonometry  Operator=tan
  Fx_rl : Outport
  Fy_rl : Outport  Port=2
  wires:
  Add/1 -> Divide/2, Divide1/2
  Subsystem/3("D ") -> Subsystem1/4(D)
  Subsystem3/2("E ") -> Subsystem2/3(E)
  Constant/1 -> Add/2
  Divide/1 -> B8/1
  Subsystem/1("B ") -> Subsystem1/2(B)
  Abs/1 -> Divide3/1
  Subsystem3/1("B ") -> Subsystem2/2(B)
  B4/1 -> Subsystem2/1("X ")
  Subsystem/2(E) -> Subsystem1/3(E)
  Fz_rl/1 -> Subsystem3/1("Fz "), Subsystem/1(FZ)
  Divide3/1 -> Product1/1
  Product1/1 -> Fy_rl/1
  SlipRate_rl/1 -> Divide/1, Add/1, B3/1
  B8/1 -> Math Function1/1, Abs1/1
  Math Function1/1 -> Add1/2
  Divide2/1 -> Product/1
  Beta_rl/1 -> Trigonometric Function/1, B4/1
  Sqrt/1 -> Divide2/2, Divide3/2
  Divide1/1 -> B1/1
  Subsystem3/3("D ") -> Subsystem2/4(D)
  B3/1 -> Subsystem1/1(X)
  Product/1 -> Fx_rl/1
  Add1/1 -> Sqrt/1
  Subsystem1/1(Fx0) -> Product/2
  Math Function/1 -> Add1/1
  Subsystem2/1(Fy0) -> Product1/2
  Trigonometric Function/1 -> Divide1/1
  Abs1/1 -> Divide2/1
  B1/1 -> Math Function/1, Abs/1

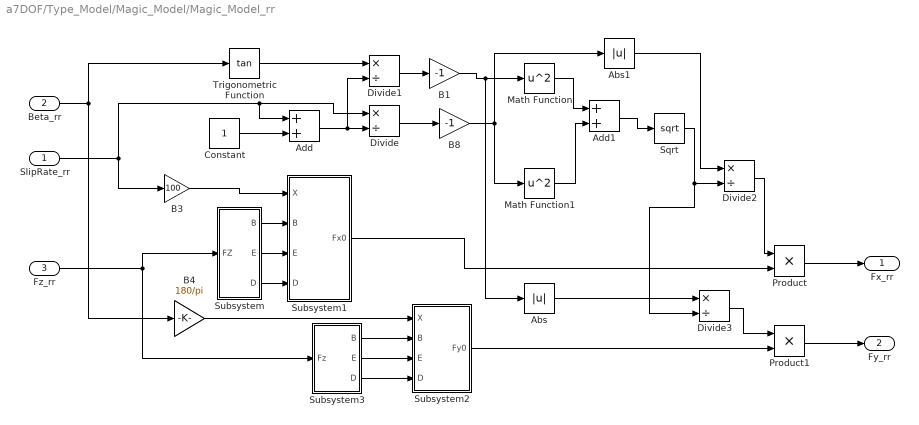
== system a7DOF/Type_Model/Magic_Model/Magic_Model_rr ==
  SlipRate_rr : Inport
  Beta_rr : Inport  Port=2
  Fz_rr : Inport  Port=3
  Abs : Abs
  Abs1 : Abs
  Add : Sum
  Add1 : Sum
  B1 : Gain  Gain=-1
  B3 : Gain  Gain=100
  B4 : Gain  Gain=180/pi
  B8 : Gain  Gain=-1
  Constant : Constant
  Divide{,1..3} (4 alike) : Product  Inputs=*/
  Math Function : Math  Operator=square  SignedPower=on  SaturateOnIntegerOverflow=on
  Math Function1 : Math  Operator=square  SignedPower=on  SaturateOnIntegerOverflow=on
  Product : Product  RndMeth=Zero
  Product1 : Product  RndMeth=Zero
  Sqrt : Sqrt  SaturateOnIntegerOverflow=on
  Subsystem : Subsystem
  Subsystem1 : Subsystem
  Subsystem2 : Subsystem
  Subsystem3 : Subsystem
  Trigonometric Function : Trigonometry  Operator=tan
  Fx_rr : Outport
  Fy_rr : Outport  Port=2
  wires:
  Product/1 -> Fx_rr/1
  SlipRate_rr/1 -> Divide/1, Add/1, B3/1
  Sqrt/1 -> Divide2/2, Divide3/2
  Divide/1 -> B8/1
  Subsystem1/1(Fx0) -> Product/2
  Divide3/1 -> Product1/1
  Subsystem/1("B ") -> Subsystem1/2(B)
  B4/1 -> Subsystem2/1("X ")
  Subsystem3/3("D ") -> Subsystem2/4(D)
  Fz_rr/1 -> Subsystem3/1("Fz "), Subsystem/1(FZ)
  Add/1 -> Divide/2, Divide1/2
  Divide2/1 -> Product/1
  Divide1/1 -> B1/1
  Constant/1 -> Add/2
  Subsystem3/2("E ") -> Subsystem2/3(E)
  Subsystem2/1(Fy0) -> Product1/2
  Subsystem3/1("B ") -> Subsystem2/2(B)
  Subsystem/3("D ") -> Subsystem1/4(D)
  Beta_rr/1 -> Trigonometric Function/1, B4/1
  B1/1 -> Math Function/1, Abs/1
  Abs/1 -> Divide3/1
  B3/1 -> Subsystem1/1(X)
  Trigonometric Function/1 -> Divide1/1
  Add1/1 -> Sqrt/1
  B8/1 -> Math Function1/1, Abs1/1
  Product1/1 -> Fy_rr/1
  Subsystem/2(E) -> Subsystem1/3(E)
  Abs1/1 -> Divide2/1
  Math Function/1 -> Add1/1
  Math Function1/1 -> Add1/2

== system a7DOF/Vehicle_Model/Subsystem/Resistance ==
  "Vx " : Inport
  A1 : Constant  Value=1/21.15
  Add5 : Sum
  Add6 : Sum
  Constant : Constant
  Constant1 : Constant  Value=0
  Gain : Gain  Gain=3.6*3.6
  Gain1 : Gain  Gain=1/1500
  Math Function : Math  Operator=square  SignedPower=on  SaturateOnIntegerOverflow=on
  Product : Product  Inputs=3
  Product10 : Product  Inputs=3  RndMeth=Zero
  Product11 : Product  RndMeth=Zero
  Product12 : Product  RndMeth=Zero
  Switch : Switch  Criteria=u2 > Threshold
  Resistance : Outport
  wires:
  Gain1/1 -> Add5/1
  Constant/1 -> Add5/2
  Switch/1 -> Add6/2
  [m] -> Product/1
  Product/1 -> Product12/2
  "Vx "/1 -> Math Function/1, Switch/2
  A1/1 -> Product10/3
  Product11/1 -> Add6/1
  Math Function/1 -> Gain1/1, Gain/1
  [A] -> Product10/2
  [Cd] -> Product10/1
  Add6/1 -> Resistance/1
  Constant1/1 -> Switch/3
  Add5/1 -> Product12/1
  Gain/1 -> Product11/1
  Product12/1 -> Switch/1
  Product10/1 -> Product11/2
  [g] -> Product/2
  [Roll_Res_Coe] -> Product/3

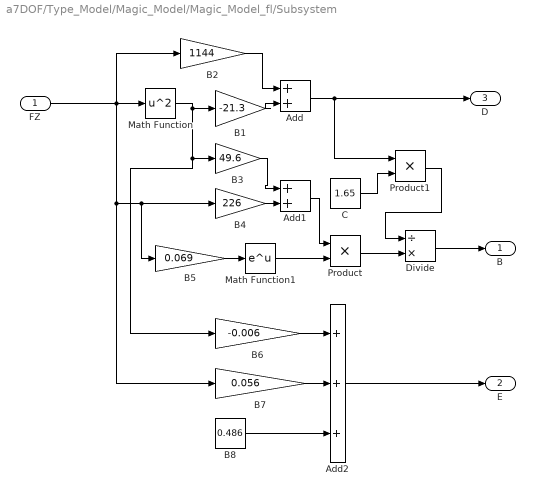
== system a7DOF/Type_Model/Magic_Model/Magic_Model_fl/Subsystem ==
  FZ : Inport
  Add : Sum
  Add1 : Sum
  Add2 : Sum  Inputs=+++
  B1 : Gain  Gain=-21.3
  B2 : Gain  Gain=1144
  B3 : Gain  Gain=49.6
  B4 : Gain  Gain=226
  B5 : Gain  Gain=0.069
  B6 : Gain  Gain=-0.006
  B7 : Gain  Gain=0.056
  "B8 " : Constant  Value=0.486
  C : Constant  Value=1.65
  Divide : Product  Inputs=/*
  Math Function : Math  Operator=square  SignedPower=on  SaturateOnIntegerOverflow=on
  Math Function1 : Math  SignedPower=on  SaturateOnIntegerOverflow=on
  Product : Product  RndMeth=Zero
  Product1 : Product  RndMeth=Zero
  "B " : Outport
  E : Outport  Port=2
  "D " : Outport  Port=3
  wires:
  Math Function1/1 -> Product/2
  C/1 -> Product1/2
  "B8 "/1 -> Add2/3
  Product/1 -> Divide/2
  Add1/1 -> Product/1
  B5/1 -> Math Function1/1
  B7/1 -> Add2/2
  Divide/1 -> "B "/1
  Add2/1 -> E/1
  B6/1 -> Add2/1
  B4/1 -> Add1/2
  B3/1 -> Add1/1
  B2/1 -> Add/1
  Add/1 -> "D "/1, Product1/1
  Product1/1 -> Divide/1
  B1/1 -> Add/2
  FZ/1 -> B4/1, B5/1, B7/1, Math Function/1, B2/1
  Math Function/1 -> B6/1, B3/1, B1/1

== system a7DOF/Type_Model/Magic_Model/Magic_Model_fl/Subsystem1 ==
  X : Inport
  B : Inport  Port=2
  E : Inport  Port=3
  D : Inport  Port=4
  Add2 : Sum
  Add3 : Sum  Inputs=+-
  Add4 : Sum  Inputs=+-
  C : Constant  Value=1.3
  Product{1..4} (4 alike) : Product  RndMeth=Zero
  Sh : Constant  Value=0
  Trigonometric Function1 : Trigonometry  Operator=atan
  Trigonometric Function2 : Trigonometry  Operator=atan
  Trigonometric Function3 : Trigonometry
  Fx0 : Outport
  wires:
  X/1 -> Add2/1
  Trigonometric Function2/1 -> Product3/1
  Add3/1 -> Product2/1
  Trigonometric Function1/1 -> Add3/2
  Product1/1 -> Trigonometric Function1/1, Add4/1, Add3/1
  Sh/1 -> Add2/2
  E/1 -> Product2/2
  B/1 -> Product1/1
  Add4/1 -> Trigonometric Function2/1
  Add2/1 -> Product1/2
  Product2/1 -> Add4/2
  D/1 -> Product4/2
  Trigonometric Function3/1 -> Product4/1
  Product4/1 -> Fx0/1
  Product3/1 -> Trigonometric Function3/1
  C/1 -> Product3/2

== system a7DOF/Type_Model/Magic_Model/Magic_Model_fl/Subsystem2 ==
  "X " : Inport
  B : Inport  Port=2
  E : Inport  Port=3
  D : Inport  Port=4
  Add3 : Sum  Inputs=+-
  Add4 : Sum  Inputs=+-
  C : Constant  Value=1.3
  Product{1..4} (4 alike) : Product  RndMeth=Zero
  Scope : Scope
  Trigonometric Function1 : Trigonometry  Operator=atan
  Trigonometric Function2 : Trigonometry  Operator=atan
  Trigonometric Function3 : Trigonometry
  Fy0 : Outport
  wires:
  Trigonometric Function2/1 -> Product3/1
  Add3/1 -> Product2/1
  Trigonometric Function1/1 -> Add3/2
  Product1/1 -> Trigonometric Function1/1, Add4/1, Add3/1
  E/1 -> Product2/2
  B/1 -> Product1/1
  Add4/1 -> Trigonometric Function2/1
  "X "/1 -> Product1/2
  Product2/1 -> Add4/2
  D/1 -> Product4/2
  Trigonometric Function3/1 -> Scope/1, Product4/1
  Product4/1 -> Fy0/1
  Product3/1 -> Trigonometric Function3/1
  C/1 -> Product3/2

== system a7DOF/Type_Model/Magic_Model/Magic_Model_fl/Subsystem3 ==
  "Fz " : Inport
  Add : Sum  Inputs=+++
  Constant : Constant  Value=1.3
  Divide : Product  Inputs=/*
  Math Function : Math  Operator=square  SignedPower=on  SaturateOnIntegerOverflow=on
  Math Function1 : Math  Operator=square  SignedPower=on  SaturateOnIntegerOverflow=on
  Product : Product  RndMeth=Zero
  Sum : Sum  Inputs=|++
  Trigonometric Function : Trigonometry  Operator=atan
  Trigonometric Function1 : Trigonometry
  a1 : Gain  Gain=-22.1
  a2 : Gain  Gain=1011
  a3 : Gain  Gain=1078
  a4 : Gain  Gain=1.82
  a5 : Gain  Gain=0.208
  a6 : Gain  Gain=0
  a7 : Gain  Gain=-0.354
  a8 : Constant  Value=0.707
  "B " : Outport
  "E " : Outport  Port=2
  "D " : Outport  Port=3
  wires:
  "Fz "/1 -> a7/1, Math Function1/1, a5/1, a2/1, Math Function/1
  Math Function/1 -> a1/1
  a1/1 -> Sum/1
  a2/1 -> Sum/2
  a5/1 -> Trigonometric Function/1
  Trigonometric Function/1 -> a4/1
  a4/1 -> Trigonometric Function1/1
  Trigonometric Function1/1 -> a3/1
  Constant/1 -> Product/1
  Sum/1 -> "D "/1, Product/2
  Product/1 -> Divide/1
  a3/1 -> Divide/2
  Divide/1 -> "B "/1
  Math Function1/1 -> a6/1
  a6/1 -> Add/1
  a7/1 -> Add/2
  a8/1 -> Add/3
  Add/1 -> "E "/1

== system a7DOF/Type_Model/Magic_Model/Magic_Model_fr/Subsystem ==
  FZ : Inport
  Add : Sum
  Add1 : Sum
  Add2 : Sum  Inputs=+++
  B1 : Gain  Gain=-21.3
  B2 : Gain  Gain=1144
  B3 : Gain  Gain=49.6
  B4 : Gain  Gain=226
  B5 : Gain  Gain=0.069
  B6 : Gain  Gain=-0.006
  B7 : Gain  Gain=0.056
  "B8 " : Constant  Value=0.486
  C : Constant  Value=1.65
  Divide : Product  Inputs=/*
  Math Function : Math  Operator=square  SignedPower=on  SaturateOnIntegerOverflow=on
  Math Function1 : Math  SignedPower=on  SaturateOnIntegerOverflow=on
  Product : Product  RndMeth=Zero
  Product1 : Product  RndMeth=Zero
  "B " : Outport
  E : Outport  Port=2
  "D " : Outport  Port=3
  wires:
  Math Function1/1 -> Product/2
  C/1 -> Product1/2
  "B8 "/1 -> Add2/3
  Product/1 -> Divide/2
  Add1/1 -> Product/1
  B5/1 -> Math Function1/1
  B7/1 -> Add2/2
  Divide/1 -> "B "/1
  Add2/1 -> E/1
  B6/1 -> Add2/1
  B4/1 -> Add1/2
  B3/1 -> Add1/1
  B2/1 -> Add/1
  Add/1 -> "D "/1, Product1/1
  Product1/1 -> Divide/1
  B1/1 -> Add/2
  FZ/1 -> B4/1, B5/1, B7/1, Math Function/1, B2/1
  Math Function/1 -> B6/1, B3/1, B1/1

== system a7DOF/Type_Model/Magic_Model/Magic_Model_fr/Subsystem1 ==
  X : Inport
  B : Inport  Port=2
  E : Inport  Port=3
  D : Inport  Port=4
  Add2 : Sum
  Add3 : Sum  Inputs=+-
  Add4 : Sum  Inputs=+-
  C : Constant  Value=1.3
  Product{1..4} (4 alike) : Product  RndMeth=Zero
  Sh : Constant  Value=0
  Trigonometric Function1 : Trigonometry  Operator=atan
  Trigonometric Function2 : Trigonometry  Operator=atan
  Trigonometric Function3 : Trigonometry
  Fx0 : Outport
  wires:
  X/1 -> Add2/1
  Trigonometric Function2/1 -> Product3/1
  Add3/1 -> Product2/1
  Trigonometric Function1/1 -> Add3/2
  Product1/1 -> Trigonometric Function1/1, Add4/1, Add3/1
  Sh/1 -> Add2/2
  E/1 -> Product2/2
  B/1 -> Product1/1
  Add4/1 -> Trigonometric Function2/1
  Add2/1 -> Product1/2
  Product2/1 -> Add4/2
  D/1 -> Product4/2
  Trigonometric Function3/1 -> Product4/1
  Product4/1 -> Fx0/1
  Product3/1 -> Trigonometric Function3/1
  C/1 -> Product3/2

== system a7DOF/Type_Model/Magic_Model/Magic_Model_fr/Subsystem2 ==
  "X " : Inport
  B : Inport  Port=2
  E : Inport  Port=3
  D : Inport  Port=4
  Add3 : Sum  Inputs=+-
  Add4 : Sum  Inputs=+-
  C : Constant  Value=1.3
  Product{1..4} (4 alike) : Product  RndMeth=Zero
  Scope : Scope
  Trigonometric Function1 : Trigonometry  Operator=atan
  Trigonometric Function2 : Trigonometry  Operator=atan
  Trigonometric Function3 : Trigonometry
  Fy0 : Outport
  wires:
  Trigonometric Function2/1 -> Product3/1
  Add3/1 -> Product2/1
  Trigonometric Function1/1 -> Add3/2
  Product1/1 -> Trigonometric Function1/1, Add4/1, Add3/1
  E/1 -> Product2/2
  B/1 -> Product1/1
  Add4/1 -> Trigonometric Function2/1
  "X "/1 -> Product1/2
  Product2/1 -> Add4/2
  D/1 -> Product4/2
  Trigonometric Function3/1 -> Scope/1, Product4/1
  Product4/1 -> Fy0/1
  Product3/1 -> Trigonometric Function3/1
  C/1 -> Product3/2

== system a7DOF/Type_Model/Magic_Model/Magic_Model_fr/Subsystem3 ==
  "Fz " : Inport
  Add : Sum  Inputs=+++
  Constant : Constant  Value=1.3
  Divide : Product  Inputs=/*
  Math Function : Math  Operator=square  SignedPower=on  SaturateOnIntegerOverflow=on
  Math Function1 : Math  Operator=square  SignedPower=on  SaturateOnIntegerOverflow=on
  Product : Product  RndMeth=Zero
  Sum : Sum  Inputs=|++
  Trigonometric Function : Trigonometry  Operator=atan
  Trigonometric Function1 : Trigonometry
  a1 : Gain  Gain=-22.1
  a2 : Gain  Gain=1011
  a3 : Gain  Gain=1078
  a4 : Gain  Gain=1.82
  a5 : Gain  Gain=0.208
  a6 : Gain  Gain=0
  a7 : Gain  Gain=-0.354
  a8 : Constant  Value=0.707
  "B " : Outport
  "E " : Outport  Port=2
  "D " : Outport  Port=3
  wires:
  "Fz "/1 -> a7/1, Math Function1/1, a5/1, a2/1, Math Function/1
  Math Function/1 -> a1/1
  a1/1 -> Sum/1
  a2/1 -> Sum/2
  a5/1 -> Trigonometric Function/1
  Trigonometric Function/1 -> a4/1
  a4/1 -> Trigonometric Function1/1
  Trigonometric Function1/1 -> a3/1
  Constant/1 -> Product/1
  Sum/1 -> "D "/1, Product/2
  Product/1 -> Divide/1
  a3/1 -> Divide/2
  Divide/1 -> "B "/1
  Math Function1/1 -> a6/1
  a6/1 -> Add/1
  a7/1 -> Add/2
  a8/1 -> Add/3
  Add/1 -> "E "/1

== system a7DOF/Type_Model/Magic_Model/Magic_Model_rl/Subsystem ==
  FZ : Inport
  Add : Sum
  Add1 : Sum
  Add2 : Sum  Inputs=+++
  B1 : Gain  Gain=-21.3
  B2 : Gain  Gain=1144
  B3 : Gain  Gain=49.6
  B4 : Gain  Gain=226
  B5 : Gain  Gain=0.069
  B6 : Gain  Gain=-0.006
  B7 : Gain  Gain=0.056
  "B8 " : Constant  Value=0.486
  C : Constant  Value=1.65
  Divide : Product  Inputs=/*
  Math Function : Math  Operator=square  SignedPower=on  SaturateOnIntegerOverflow=on
  Math Function1 : Math  SignedPower=on  SaturateOnIntegerOverflow=on
  Product : Product  RndMeth=Zero
  Product1 : Product  RndMeth=Zero
  "B " : Outport
  E : Outport  Port=2
  "D " : Outport  Port=3
  wires:
  Math Function/1 -> B1/1, B3/1, B6/1
  FZ/1 -> B2/1, Math Function/1, B7/1, B5/1, B4/1
  B1/1 -> Add/2
  Product1/1 -> Divide/1
  Add/1 -> Product1/1, "D "/1
  B2/1 -> Add/1
  B3/1 -> Add1/1
  B4/1 -> Add1/2
  B6/1 -> Add2/1
  Add2/1 -> E/1
  Divide/1 -> "B "/1
  B7/1 -> Add2/2
  B5/1 -> Math Function1/1
  Add1/1 -> Product/1
  Product/1 -> Divide/2
  "B8 "/1 -> Add2/3
  C/1 -> Product1/2
  Math Function1/1 -> Product/2

== system a7DOF/Type_Model/Magic_Model/Magic_Model_rl/Subsystem1 ==
  X : Inport
  B : Inport  Port=2
  E : Inport  Port=3
  D : Inport  Port=4
  Add2 : Sum
  Add3 : Sum  Inputs=+-
  Add4 : Sum  Inputs=+-
  C : Constant  Value=1.3
  Product{1..4} (4 alike) : Product  RndMeth=Zero
  Sh : Constant  Value=0
  Trigonometric Function1 : Trigonometry  Operator=atan
  Trigonometric Function2 : Trigonometry  Operator=atan
  Trigonometric Function3 : Trigonometry
  Fx0 : Outport
  wires:
  C/1 -> Product3/2
  Product3/1 -> Trigonometric Function3/1
  Product4/1 -> Fx0/1
  Trigonometric Function3/1 -> Product4/1
  D/1 -> Product4/2
  Product2/1 -> Add4/2
  Add2/1 -> Product1/2
  Add4/1 -> Trigonometric Function2/1
  B/1 -> Product1/1
  E/1 -> Product2/2
  Sh/1 -> Add2/2
  Product1/1 -> Add3/1, Add4/1, Trigonometric Function1/1
  Trigonometric Function1/1 -> Add3/2
  Add3/1 -> Product2/1
  Trigonometric Function2/1 -> Product3/1
  X/1 -> Add2/1

== system a7DOF/Type_Model/Magic_Model/Magic_Model_rl/Subsystem2 ==
  "X " : Inport
  B : Inport  Port=2
  E : Inport  Port=3
  D : Inport  Port=4
  Add3 : Sum  Inputs=+-
  Add4 : Sum  Inputs=+-
  C : Constant  Value=1.3
  Product{1..4} (4 alike) : Product  RndMeth=Zero
  Scope : Scope
  Trigonometric Function1 : Trigonometry  Operator=atan
  Trigonometric Function2 : Trigonometry  Operator=atan
  Trigonometric Function3 : Trigonometry
  Fy0 : Outport
  wires:
  C/1 -> Product3/2
  Product3/1 -> Trigonometric Function3/1
  Product4/1 -> Fy0/1
  Trigonometric Function3/1 -> Product4/1, Scope/1
  D/1 -> Product4/2
  Product2/1 -> Add4/2
  "X "/1 -> Product1/2
  Add4/1 -> Trigonometric Function2/1
  B/1 -> Product1/1
  E/1 -> Product2/2
  Product1/1 -> Add3/1, Add4/1, Trigonometric Function1/1
  Trigonometric Function1/1 -> Add3/2
  Add3/1 -> Product2/1
  Trigonometric Function2/1 -> Product3/1
